simulink model "single_NMM_Adaptive_Controller"  (R2019a)
settings: Solver=ode4  StartTime=0.0  StopTime=10  RelTol=1e-3
PostLoadFcn:
  | ButtonName = questdlg(['Today is ' date newline 'Have a Nice Day' newline...
  |  'The Simulink model was created by Lige on 25-Dec-2019'...
  | newline 'The Author''s Email is lige960103@gmail.com',newline,newline,newline,...
  | 'Would you want the dialog box to be shown when the file is opened again? '], ...
  | 'Open Question', ...
  | 'Yes', 'No', 'Yes');
  | if strcmp(ButtonName,'No')
  | set_param(gcs,'PostLoadFcn','')
  | save_system(gcs)
  | end
  | clear ButtonName
StopFcn:
  | fi=get_param([bdroot '/Show/ref_out'],'Commented');
  | if strcmp(fi,'off')
  | plot(ref_out.Time,ref_out.Data(:,1),ref_out.Time,ref_out.Data(:,2))
  | legend('ref','out')
  | ylabel('y (mV)')
  | xlabel('t')
  | title('Output and Reference')
  | end
  | 
  | fi=get_param([bdroot '/Show/err'],'Commented');
  | if strcmp(fi,'off')
  | figure;
  | plot(err.Time,err.Data)
  | legend('error')
  | ylabel('value (mV)')
  | xlabel('t (s)')
  | title('Tracking Error')
  | end
  | 
  | fi=get_param([bdroot '/Show/Hat_A_and_A'],'Commented');
  | if strcmp(fi,'off')
  | figure;
  | plot(Hat_A_and_A.Time,Hat_A_and_A.Data(:,1),Hat_A_and_A.Time,Hat_A_and_A.Data(:,2))
  | legend('hat A ','A')
  | ylabel('value (mV)')
  | xlabel('t (s)')
  | title('Parameters Estimated')
  | end
  | 
  | fi=get_param([bdroot '/Show/u'],'Commented');
  | if strcmp(fi,'off')
  | figure;
  | plot(u.Time,u.Data)
  | legend('u')
  | ylabel('value (mV)')
  | xlabel('t (s)')
  | title('Control Input')
  | end
undefined symbols (not defined in the file): Single_NMM_Parameters
libraries: simulink x2
settings Model: Creator=Administrator  LastModifiedBy=liuxian
settings DataIOCC: SaveOutput=off  SignalLogging=off  DSMLogging=off  SaveTime=off  ReturnWorkspaceOutputs=off
settings OptimizationCC: DefaultParameterBehavior=Inlined  EnhancedBackFolding=on  PassReuseOutputArgsAs=Individual arguments  OptimizeBlockOrder=speed  DifferentSizesBufferReuse=on  OptimizationCustomize=off
settings DebuggingCC: ParameterTunabilityLossMsg=error
settings SFSimCC: MATLABDynamicMemAlloc=off
settings RTWCC: SystemTargetFile=ert.tlc  TemplateMakefile=ert_default_tmf  GenerateReport=on  IncludeHyperlinkInReport=on  LaunchReport=on  GenerateTraceInfo=on  GenerateTraceReport=on  GenerateTraceReportSl=on  GenerateTraceReportSf=on  GenerateTraceReportEml=on
settings CodeAppCC: ForceParamTrailComments=on  IgnoreCustomStorageClasses=off  OperatorAnnotations=on  SimulinkDataObjDesc=on  SFDataObjDesc=on  InsertBlockDesc=on
settings ERTTargetCC: TargetLangStandard=C99 (ISO)  GenerateSampleERTMain=on  MatFileLogging=on  SupportContinuousTime=on  InlinedParameterPlacement=NonHierarchical  ERTCustomFileTemplate=example_file_process.tlc  ERTFilePackagingFormat=CompactWithDataFile

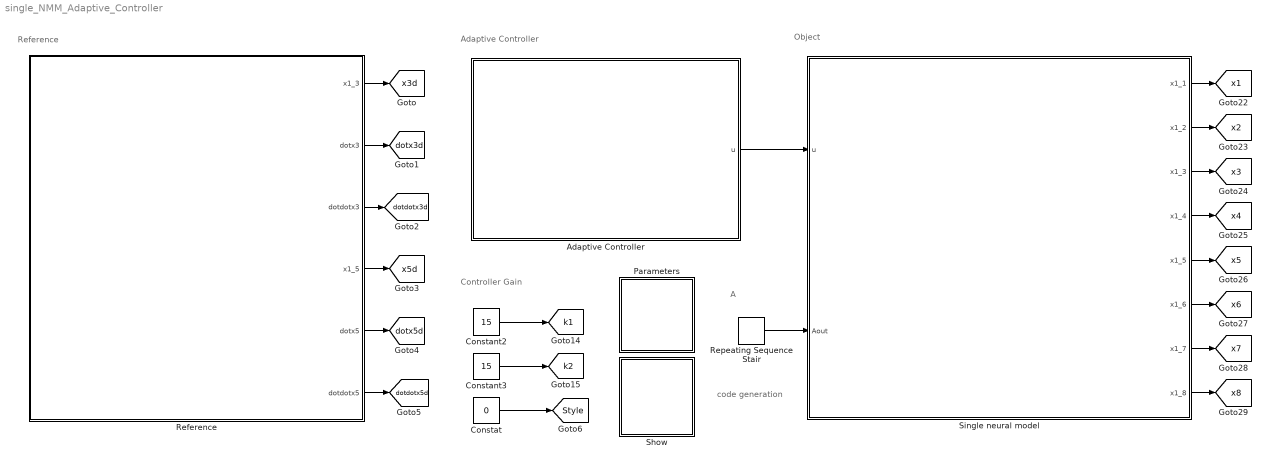
== system single_NMM_Adaptive_Controller ==
  note: code
      | generation
  note: Controller Gain
  note: Adaptive Controller
  note: Reference
  note: Object
  note: A
  Adaptive Controller : Subsystem
      settings: RTWSystemCode=Nonreusable function  RTWFcnNameOpts=Use subsystem name
      mask Display: disp('Adaptive Controller')
  Constant2 : Constant  Value=15
  Constant3 : Constant  Value=15
  Constat : Constant  Value=0  OutDataTypeStr=boolean
  Parameters : Subsystem
      mask Display: disp('Param')
  Reference : Subsystem  mask(Reference  model){AA=Single_NMM_Parameters.Normal_A, B=Single_NMM_Parameters.B, a=Single_NMM_Parameters.a, b1=Single_NMM_Parameters.b, C_1=Single_NMM_Parameters.C1, C_2=Single_NMM_Parameters.C2, C_3=Single_NMM_Parameters.C3, C_4=Single_NMM_Parameters.C4, r=Single_NMM_Parameters.r, e_0=Single_NMM_Parameters.e_0, v_0=Single_NMM_Parameters.v_0, a_d=Single_NMM_Parameters.a_d, SimpleTime=Single_NMM_Parameters.simple_time}
      mask prompts: AA "A"; b1 "b"; C_1 "C1"; C_2 "C2"; C_3 "C3"; C_4 "C4"; e_0 "e0"; v_0 "v0"; a_d "ad"; SimpleTime "Simple Time of P(t)"
      mask help: The block is the mask of the neural mass model (NMM). The parameters(A and B) are average gain, and the parameter A will result in different model output. The parameters (a, a_d and b) is time constant. The parameter (C1-C4) are average number. Three parameters (v_0, e_0 anf r) define a nonlinear function named sigmoid function.
      settings: RTWSystemCode=Nonreusable function  RTWFcnNameOpts=Use subsystem name
      mask Display:
      | port_label('output',1,'x3')
      | port_label('output',2,'dotx3')
      | port_label('output',3,'dotdotx3')
      | port_label('output',4,'x5')
      | port_label('output',5,'dotx5')
      | port_label('output',6,'dotdotx5')
      | disp('Reference Normal Single NMM')
  Repeating Sequence Stair : simulink/Sources/Repeating Sequence Stair  OutValues=[3.25 3.4 3.5 3.6 3.4 ].'  tsamp=2  OutMin=[]  OutMax=[]  OutDataTypeStr=double  OutputDataTypeScalingMode=double  OutDataType=fixdt(0,8)  ConRadixGroup=Best Precision: Vector-wise  OutScaling=2^-12
  Show : Subsystem
      mask Display: disp('Show')
  Single neural model : Subsystem  mask(Mask Single neural model by lige){A_status=off, AA=Single_NMM_Parameters.Abnormal_A, B=Single_NMM_Parameters.B, a=Single_NMM_Parameters.a, b1=Single_NMM_Parameters.b, C_1=Single_NMM_Parameters.C1, C_2=Single_NMM_Parameters.C2, C_3=Single_NMM_Parameters.C3, C_4=Single_NMM_Parameters.C4, r=Single_NMM_Parameters.r, e_0=Single_NMM_Parameters.e_0, v_0=Single_NMM_Parameters.v_0, a_d=Single_NMM_Parameters.a_d, SimpleTime=Single_NMM_Parameters.simple_time}
      mask prompts: A_status "Change A in GUI or input"; AA "A"; b1 "b"; C_1 "C1"; C_2 "C2"; C_3 "C3"; C_4 "C4"; e_0 "e0"; v_0 "v0"; a_d "ad"; SimpleTime "Simple Time of P(t)"
      mask help: The block is the mask of the neural mass model (NMM). The parameters(A and B) are average gain, and the parameter A will result in different model output. The parameters (a, a_d and b) is time constant. The parameter (C1-C4) are average number. Three parameters (v_0, e_0 anf r) define a nonlinear function named sigmoid function.
      settings: RTWSystemCode=Nonreusable function  RTWFcnNameOpts=Use subsystem name
      mask Callback A_status:
      | A_s=get(gcbh,'A_status');
      | block_name=gcb;
      | A_vis=get(gcbh,'MaskVisibilities');
      | str=['port_label(''input'',1,''u'');'...
      | 'port_label(''input'',2,''The port is unvalid'');'...
      | 'port_label(''output'',1,''x_1'');'...
      | 'port_label(''output'',2,''x_2'');'...
      | 'port_label(''output'',3,''x_3'');'...
      | 'port_label(''output'',4,''x_4'');'...
      | 'port_label(''output'',5,''x_5'');'...
      | 'port_label(''output'',6,''x_6'');'...
      | 'port_label(''output'',7,''x_7'');'...
      | 'port_label(''output'',8,''x_8'');disp(''Single NMM'')'];
      | str1=['port_label(''input'',1,''u'');'...
      | 'port_label(''input'',2,''A'');'...
      | 'port_label(''output'',1,''x_1'');'...
      | 'port_label(''output'',2,''x_2'');'...
      | 'port_label(''output'',3,''x_3'');'...
      | 'port_label(''output'',4,''x_4'');'...
      | 'port_label(''output'',5,''x_5'');'...
      | 'port_label(''output'',6,''x_6'');'...
      | 'port_label(''output'',7,''x_7'');'...
      | 'port_label(''output'',8,''x_8'');disp(''Single NMM'')'];
      | if strcmp(A_s,'on')
      |     set(gcbh,'MaskDisplay',str)
      |     A_vis{2}='on';
      |     set_param([block_name '/gain'],'Gain','1');
      |     set_param([block_name '/gaout'],'Gain','0');
      | else
      |     set(gcbh,'MaskDisplay',str1)
      |     A_vis{2}='off';
      |     set_param([block_name '/gain'],'Gain','0');
      |     set_param([block_name '/gaout'],'Gain','1');
      | end
      | set(gcbh,'MaskVisibilities',A_vis)
      mask Display: port_label('input',1,'u');port_label('input',2,'A');port_label('output',1,'x_1');port_label('output',2,'x_2');port_label('output',3,'x_3');port_label('output',4,'x_4');port_label('output',5,'x_5');port_label('output',6,'x_6');port_label('output',7,'x_7');port_label('output',8,'x_8');disp('Single NMM')
  tag scope: Style=global, dotdotx3d=global, dotdotx5d=global, dotx3d=global, dotx5d=global, k1=global, k2=global, x1=global, x2=global, x3=global, x3d=global, x4=global, x5=global, x5d=global, x6=global, x7=global, x8=global
  wires:
  Repeating Sequence Stair/1 -> Single neural model/2(Aout)
  Single neural model/1(x1_1) -> [x1]
  Single neural model/2(x1_2) -> [x2]
  Single neural model/3(x1_3) -> [x3]
  Single neural model/4(x1_4) -> [x4]
  Single neural model/5(x1_5) -> [x5]
  Single neural model/6(x1_6) -> [x6]
  Single neural model/7(x1_7) -> [x7]
  Single neural model/8(x1_8) -> [x8]
  Reference/3(dotdotx3) -> [dotdotx3d]
  Reference/1(x1_3) -> [x3d]
  Reference/2(dotx3) -> [dotx3d]
  Reference/4(x1_5) -> [x5d]
  Reference/5(dotx5) -> [dotx5d]
  Reference/6(dotdotx5) -> [dotdotx5d]
  Constant2/1 -> [k1]
  Constant3/1 -> [k2]
  Adaptive Controller/1(u) -> Single neural model/1(u)
  Constat/1 -> [Style]

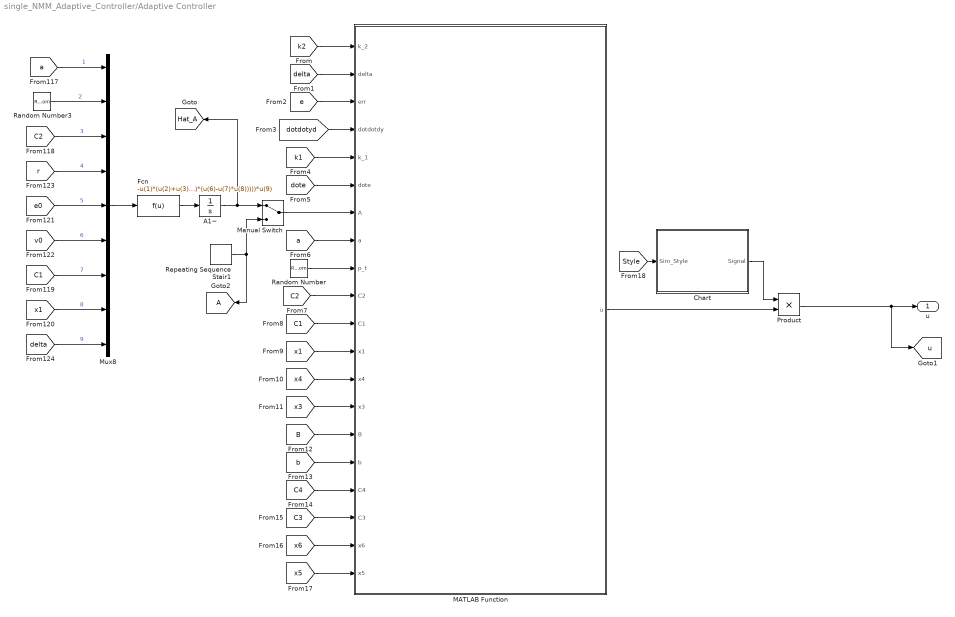
== system single_NMM_Adaptive_Controller/Adaptive Controller ==
  A1~ : Integrator  InitialCondition=3  LimitOutput=on  UpperSaturationLimit=6  LowerSaturationLimit=2
  Chart : Stateflow chart  BlockKeywords=__PRM__SERIALIZED__DATA__:Stateflow Chart,Stateflow Diagram  TreatAsAtomicUnit=on
  Fcn : Fcn  Expr=-u(1)*(u(2)+u(3)*2*u(5)/(1+exp(u(4)*(u(6)-u(7)*u(8)))))*u(9)
  MATLAB Function : MATLAB Function  TreatAsAtomicUnit=on
  Manual Switch : ManualSwitch
  Mux8 : Mux  Inputs=9
  Product : Product
  Random Number : RandomNumber  Mean=90  Variance=30  SampleTime=Single_NMM_Parameters.simple_time
  Random Number3 : RandomNumber  Mean=90  Variance=30  SampleTime=Single_NMM_Parameters.simple_time
  Repeating Sequence Stair1 : simulink/Sources/Repeating Sequence Stair  OutValues=[3.25 3.4 3.5 3.6 3.4 ].'  tsamp=2  OutMin=[]  OutMax=[]  OutDataTypeStr=double  OutputDataTypeScalingMode=double  OutDataType=fixdt(0,8)  ConRadixGroup=Best Precision: Vector-wise  OutScaling=2^-12
  u : Outport
  tag scope: A=global, Hat_A=global, u=global
  wires:
  [x3] -> MATLAB Function/14(x3)
  [C1] -> Mux8/7  "7"
  [v0] -> Mux8/6  "6"
  Repeating Sequence Stair1/1 -> Manual Switch/2, [A]
  Fcn/1 -> A1~/1
  [a] -> MATLAB Function/8(a)
  [k1] -> MATLAB Function/5(k_1)
  [C3] -> MATLAB Function/18(C3)
  A1~/1 -> [Hat_A], Manual Switch/1
  [r] -> Mux8/4  "4"
  [e] -> MATLAB Function/3(err)
  Mux8/1 -> Fcn/1
  [b] -> MATLAB Function/16(b)
  Random Number3/1 -> Mux8/2  "2"
  [x1] -> MATLAB Function/12(x1)
  [k2] -> MATLAB Function/1(k_2)
  [C1] -> MATLAB Function/11(C1)
  [e0] -> Mux8/5  "5"
  [x6] -> MATLAB Function/19(x6)
  [dotdotyd] -> MATLAB Function/4(dotdotdy)
  [delta] -> MATLAB Function/2(delta)
  [a] -> Mux8/1  "1"
  [C2] -> Mux8/3  "3"
  [C2] -> MATLAB Function/10(C2)
  [dote] -> MATLAB Function/6(dote)
  Manual Switch/1 -> MATLAB Function/7(A)
  [C4] -> MATLAB Function/17(C4)
  [x5] -> MATLAB Function/20(x5)
  Product/1 -> [u], u/1
  [x1] -> Mux8/8  "8"
  [delta] -> Mux8/9  "9"
  [B] -> MATLAB Function/15(B)
  Random Number/1 -> MATLAB Function/9(p_t)
  [x4] -> MATLAB Function/13(x4)
  Chart/1(Signal) -> Product/1
  MATLAB Function/1(u) -> Product/2
  [Style] -> Chart/1(Sim_Style)

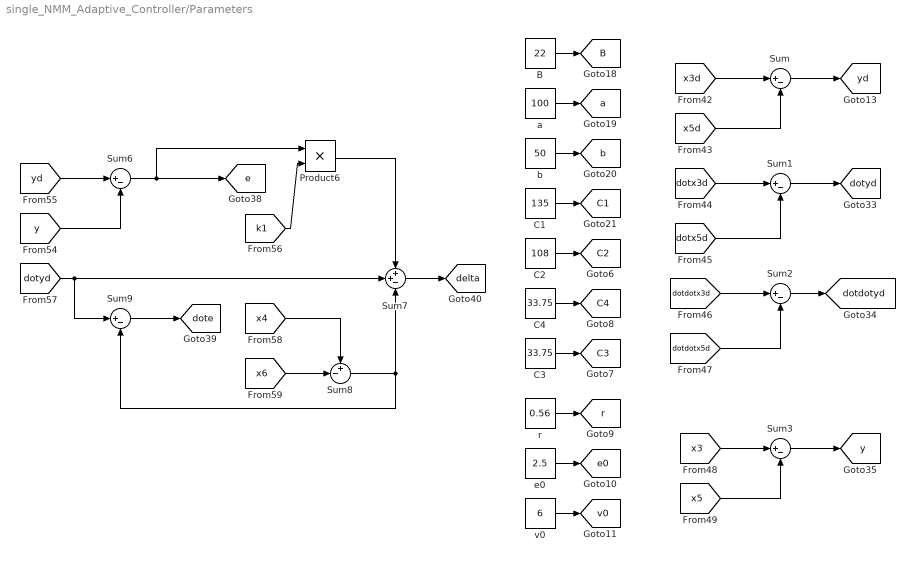
== system single_NMM_Adaptive_Controller/Parameters ==
  B : Constant  Value=22
  C1 : Constant  Value=135
  C2 : Constant  Value=108
  C3 : Constant  Value=33.75
  C4 : Constant  Value=33.75
  Product6 : Product
  Sum{,1..3,6,9} (6 alike) : Sum  Inputs=|+-
  Sum7 : Sum  Inputs=++-
  Sum8 : Sum  Inputs=+-|
  a : Constant  Value=100
  b : Constant  Value=50
  e0 : Constant  Value=2.5
  r : Constant  Value=0.56
  v0 : Constant  Value=6
  tag scope: B=global, C1=global, C2=global, C3=global, C4=global, a=global, b=global, delta=global, dotdotyd=global, dote=global, dotyd=global, e0=global, e=global, r=global, v0=global, y=global, yd=global
  wires:
  [dotx3d] -> Sum1/1
  [dotdotx5d] -> Sum2/2
  Sum9/1 -> [dote]
  [dotx5d] -> Sum1/2
  B/1 -> [B]
  e0/1 -> [e0]
  C2/1 -> [C2]
  [yd] -> Sum6/1
  [dotyd] -> Sum9/1, Sum7/2
  Sum7/1 -> [delta]
  Sum1/1 -> [dotyd]
  a/1 -> [a]
  [dotdotx3d] -> Sum2/1
  Sum/1 -> [yd]
  [k1] -> Product6/2
  Sum6/1 -> Product6/1, [e]
  r/1 -> [r]
  [x5d] -> Sum/2
  Sum8/1 -> Sum7/3, Sum9/2
  C3/1 -> [C3]
  b/1 -> [b]
  [x4] -> Sum8/1
  C4/1 -> [C4]
  [y] -> Sum6/2
  [x3] -> Sum3/1
  Sum2/1 -> [dotdotyd]
  [x6] -> Sum8/2
  Sum3/1 -> [y]
  C1/1 -> [C1]
  v0/1 -> [v0]
  [x5] -> Sum3/2
  Product6/1 -> Sum7/1
  [x3d] -> Sum/1

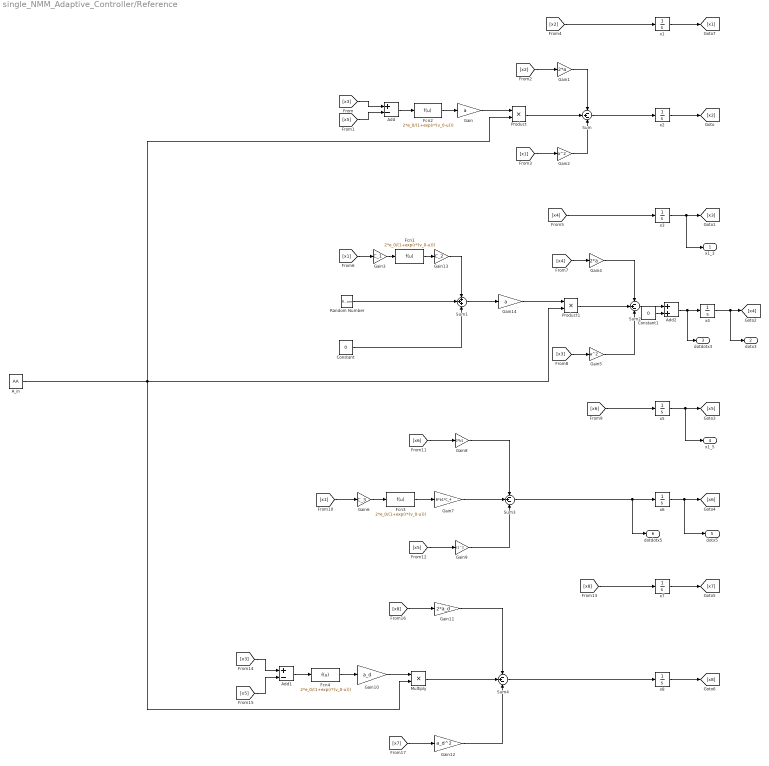
== system single_NMM_Adaptive_Controller/Reference ==
  A_in : Constant  Value=AA
  Add : Sum  Inputs=+-
  Add1 : Sum  Inputs=+-
  Add2 : Sum
  Constant : Constant  Value=0
  Constant1 : Constant  Value=0
  Fcn{1..4} (4 alike) : Fcn  Expr=2*e_0/(1+exp(r*(v_0-u)))
  Gain : Gain  Gain=a
  Gain1 : Gain  Gain=2*a
  Gain10 : Gain  Gain=a_d
  Gain11 : Gain  Gain=2*a_d
  Gain12 : Gain  Gain=a_d^2
  Gain13 : Gain  Gain=C_2
  Gain14 : Gain  Gain=a
  Gain2 : Gain  Gain=a^2
  Gain3 : Gain  Gain=C_1
  Gain4 : Gain  Gain=2*a
  Gain5 : Gain  Gain=a^2
  Gain6 : Gain  Gain=C_3
  Gain7 : Gain  Gain=B*b1*C_4
  Gain8 : Gain  Gain=2*b1
  Gain9 : Gain  Gain=b1^2
  Multiply : Product
  Product : Product
  Product1 : Product
  Random Number : RandomNumber  Mean=90  Variance=30  SampleTime=SimpleTime
  Sum{,2..4} (4 alike) : Sum  Inputs=-+-
  Sum1 : Sum  Inputs=3
  x{1..8} (8 alike) : Integrator
  x1_3 : Outport
  dotx3 : Outport  Port=2
  dotdotx3 : Outport  Port=3
  x1_5 : Outport  Port=4
  dotx5 : Outport  Port=5
  dotdotx5 : Outport  Port=6
  wires:
  Gain/1 -> Product/1
  Gain12/1 -> Sum4/3
  Gain2/1 -> Sum/3
  Random Number/1 -> Sum1/2
  Gain11/1 -> Sum4/1
  [x5] -> Add1/2
  [x1] -> Gain6/1
  Gain13/1 -> Sum1/1
  [x6] -> Gain8/1
  [x6] -> x5/1
  [x3] -> Gain5/1
  Sum/1 -> x2/1
  [x1] -> Gain2/1
  [x4] -> Gain4/1
  Sum2/1 -> Add2/1
  Fcn3/1 -> Gain7/1
  [x8] -> x7/1
  A_in/1 -> Product/2, Multiply/2, Product1/2
  [x2] -> Gain1/1
  Multiply/1 -> Sum4/2
  Gain8/1 -> Sum3/1
  [x2] -> x1/1
  Product1/1 -> Sum2/2
  Gain14/1 -> Product1/1
  Gain6/1 -> Fcn3/1
  Product/1 -> Sum/2
  Add/1 -> Fcn2/1
  Gain9/1 -> Sum3/3
  x5/1 -> [x5], x1_5/1
  [x4] -> x3/1
  x3/1 -> [x3], x1_3/1
  [x3] -> Add/1
  [x8] -> Gain11/1
  Fcn1/1 -> Gain13/1
  [x5] -> Add/2
  Gain5/1 -> Sum2/3
  [x3] -> Add1/1
  Gain7/1 -> Sum3/2
  Add1/1 -> Fcn4/1
  [x5] -> Gain9/1
  [x7] -> Gain12/1
  Sum3/1 -> dotdotx5/1, x6/1
  x1/1 -> [x1]
  x6/1 -> [x6], dotx5/1
  Gain1/1 -> Sum/1
  [x1] -> Gain3/1
  Gain4/1 -> Sum2/1
  x2/1 -> [x2]
  Fcn2/1 -> Gain/1
  Add2/1 -> dotdotx3/1, x4/1
  x4/1 -> [x4], dotx3/1
  x8/1 -> [x8]
  x7/1 -> [x7]
  Gain10/1 -> Multiply/1
  Gain3/1 -> Fcn1/1
  Sum1/1 -> Gain14/1
  Sum4/1 -> x8/1
  Constant1/1 -> Add2/2
  Constant/1 -> Sum1/3
  Fcn4/1 -> Gain10/1

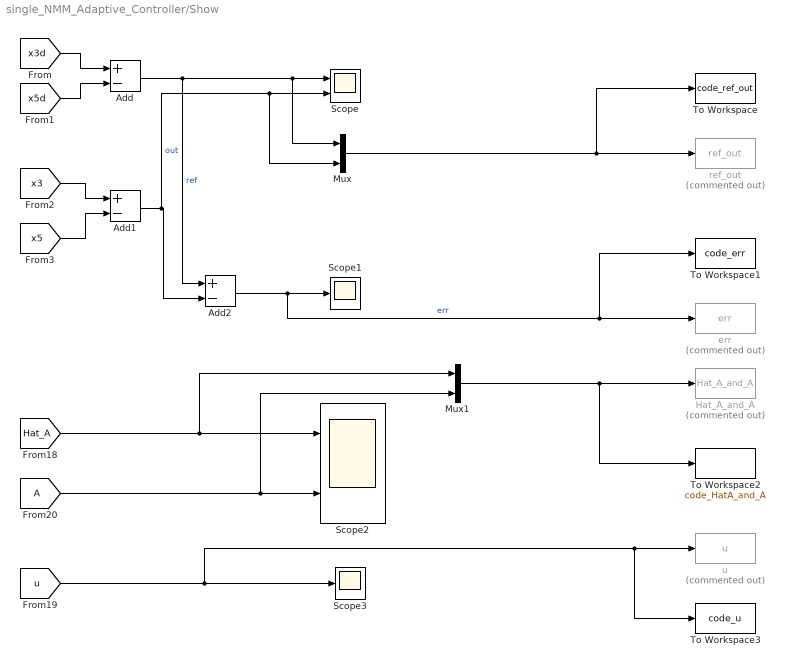
== system single_NMM_Adaptive_Controller/Show ==
  Add : Sum  Inputs=+-
  Add1 : Sum  Inputs=+-
  Add2 : Sum  Inputs=+-
  Hat_A_and_A : ToWorkspace  Commented=on  VariableName=Hat_A_and_A  SaveFormat=Timeseries  SampleTime=-1
  Mux : Mux  Inputs=2
  Mux1 : Mux  Inputs=2
  Scope : Scope  NumInputPorts=2
  Scope1 : Scope
  Scope2 : Scope  NumInputPorts=2
  Scope3 : Scope
  To Workspace : ToWorkspace  VariableName=code_ref_out  SaveFormat=Structure With Time  SampleTime=-1
  To Workspace1 : ToWorkspace  VariableName=code_err  SaveFormat=Structure With Time  SampleTime=-1
  To Workspace2 : ToWorkspace  VariableName=code_HatA_and_A  SaveFormat=Structure With Time  SampleTime=-1
  To Workspace3 : ToWorkspace  VariableName=code_u  SaveFormat=Structure With Time  SampleTime=-1
  err : ToWorkspace  Commented=on  VariableName=err  SaveFormat=Timeseries  SampleTime=-1
  ref_out : ToWorkspace  Commented=on  VariableName=ref_out  SaveFormat=Timeseries  SampleTime=-1
  u : ToWorkspace  Commented=on  VariableName=u  SaveFormat=Timeseries  SampleTime=-1
  wires:
  [x3d] -> Add/1
  [x5d] -> Add/2
  [x3] -> Add1/1
  [x5] -> Add1/2
  Add1/1 -> Mux/2, Scope/2, Add2/2  "out"
  Add/1 -> Add2/1, Mux/1, Scope/1  "ref"
  Add2/1 -> err/1, To Workspace1/1, Scope1/1  "err"
  [Hat_A] -> Mux1/1, Scope2/1
  [A] -> Mux1/2, Scope2/2
  Mux1/1 -> Hat_A_and_A/1, To Workspace2/1
  Mux/1 -> To Workspace/1, ref_out/1
  [u] -> To Workspace3/1, u/1, Scope3/1

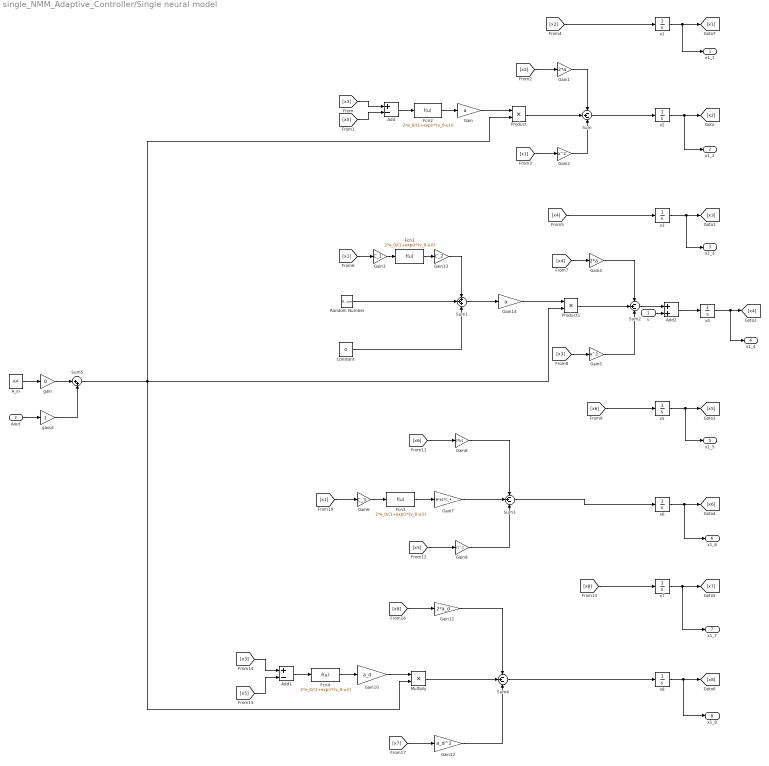
== system single_NMM_Adaptive_Controller/Single neural model ==
  u : Inport
  Aout : Inport  Port=2
  A_in : Constant  Value=AA
  Add : Sum  Inputs=+-
  Add1 : Sum  Inputs=+-
  Add2 : Sum
  Constant : Constant  Value=0
  Fcn{1..4} (4 alike) : Fcn  Expr=2*e_0/(1+exp(r*(v_0-u)))
  Gain : Gain  Gain=a
  Gain1 : Gain  Gain=2*a
  Gain10 : Gain  Gain=a_d
  Gain11 : Gain  Gain=2*a_d
  Gain12 : Gain  Gain=a_d^2
  Gain13 : Gain  Gain=C_2
  Gain14 : Gain  Gain=a
  Gain2 : Gain  Gain=a^2
  Gain3 : Gain  Gain=C_1
  Gain4 : Gain  Gain=2*a
  Gain5 : Gain  Gain=a^2
  Gain6 : Gain  Gain=C_3
  Gain7 : Gain  Gain=B*b1*C_4
  Gain8 : Gain  Gain=2*b1
  Gain9 : Gain  Gain=b1^2
  Multiply : Product
  Product : Product
  Product1 : Product
  Random Number : RandomNumber  Mean=90  Variance=30  SampleTime=SimpleTime
  Sum{,2..4} (4 alike) : Sum  Inputs=-+-
  Sum1 : Sum  Inputs=3
  Sum5 : Sum  Inputs=|++
  gain : Gain  Gain=0
  gaout : Gain
  x{1..8} (8 alike) : Integrator
  x1_1 : Outport
  x1_2 : Outport  Port=2
  x1_3 : Outport  Port=3
  x1_4 : Outport  Port=4
  x1_5 : Outport  Port=5
  x1_6 : Outport  Port=6
  x1_7 : Outport  Port=7
  x1_8 : Outport  Port=8
  wires:
  gaout/1 -> Sum5/2
  gain/1 -> Sum5/1
  A_in/1 -> gain/1
  Aout/1 -> gaout/1
  Sum5/1 -> Product1/2, Multiply/2, Product/2
  Gain10/1 -> Multiply/1
  Multiply/1 -> Sum4/2
  Gain14/1 -> Product1/1
  Product1/1 -> Sum2/2
  Product/1 -> Sum/2
  Gain/1 -> Product/1
  Sum4/1 -> x8/1
  x7/1 -> x1_7/1, [x7]
  [x1] -> Gain6/1
  Gain9/1 -> Sum3/3
  Gain11/1 -> Sum4/1
  Gain13/1 -> Sum1/1
  [x6] -> x5/1
  [x6] -> Gain8/1
  Add/1 -> Fcn2/1
  [x3] -> Gain5/1
  x8/1 -> x1_8/1, [x8]
  Sum/1 -> x2/1
  x4/1 -> x1_4/1, [x4]
  Gain3/1 -> Fcn1/1
  Sum1/1 -> Gain14/1
  Gain5/1 -> Sum2/3
  [x2] -> x1/1
  x5/1 -> x1_5/1, [x5]
  [x5] -> Add/2
  Gain12/1 -> Sum4/3
  x2/1 -> x1_2/1, [x2]
  [x8] -> Gain11/1
  Fcn1/1 -> Gain13/1
  [x3] -> Add/1
  [x8] -> x7/1
  [x1] -> Gain3/1
  Gain4/1 -> Sum2/1
  [x7] -> Gain12/1
  [x4] -> Gain4/1
  Gain2/1 -> Sum/3
  [x2] -> Gain1/1
  x3/1 -> x1_3/1, [x3]
  [x5] -> Gain9/1
  Random Number/1 -> Sum1/2
  x6/1 -> x1_6/1, [x6]
  Gain1/1 -> Sum/1
  Gain7/1 -> Sum3/2
  x1/1 -> x1_1/1, [x1]
  Fcn3/1 -> Gain7/1
  [x4] -> x3/1
  [x1] -> Gain2/1
  Fcn2/1 -> Gain/1
  Gain8/1 -> Sum3/1
  Gain6/1 -> Fcn3/1
  [x5] -> Add1/2
  Constant/1 -> Sum1/3
  [x3] -> Add1/1
  Add2/1 -> x4/1
  Sum2/1 -> Add2/1
  u/1 -> Add2/2
  Sum3/1 -> x6/1
  Add1/1 -> Fcn4/1
  Fcn4/1 -> Gain10/1

== matlab function single_NMM_Adaptive_Controller/Adaptive Controller/MATLAB Function ==
  data: k_2 input; u output; delta input; err input; dotdotdy input; k_1 input; dote input; A input; a input; p_t input; C2 input; C1 input; x1 input; x4 input; x3 input; B input; b input; C4 input; C3 input; x6 input; x5 input
function u = adptive_controller(k_2,delta,err,dotdotdy,k_1,dote,A,a,p_t,C2,C1,x1,x4,x3,B,b,C4,C3,x6,x5)
%codergen
u=k_2*delta+err+dotdotdy+k_1*dote-A*a*(p_t+C2*2*2.5/(1+exp(0.56*(6-C1*x1))))...
    +2*a*x4+a^2*x3+B*b*C4*2*2.5/(1+exp(0.56*(6-C3*x1)))-2*b*x6-b^2*x5;

== stateflow chart single_NMM_Adaptive_Controller/Adaptive Controller/Chart ==
  state All
    en:
    Signal = true;
  state Uncontroll
    en:
    Signal=false;
  state Controll
    en:
    Signal = true;
  state Uncontroll1
    en:
    Signal=false;
  state Controll1
    en:
    Signal = true;
  state Uncontroll2
    en:
    Signal=false;
  state Controll4
    en:
    Signal = true;
  state Uncontroll4
    en:
    Signal=false;
  state Controll3
    en:
    Signal = true;
  state Uncontroll3
    en:
    Signal=false;
  state Controll2
    en:
    Signal = true;
  (default) -> Uncontroll [order 1] : [Sim_Style == 0]
  (default) -> All [order 2]
  Uncontroll1 -> Controll1 : after(0.815,sec)
  Uncontroll -> Controll : after(1.1,sec)
  Controll -> Uncontroll1 : after(0.9,sec)
  Controll1 -> Uncontroll2 : after(1.185,sec)
  Uncontroll2 -> Controll2 : after(0.831,sec)
  Uncontroll4 -> Controll4 : after(1.031,sec)
  Controll2 -> Uncontroll3 : after(1.169,sec)
  Controll3 -> Uncontroll4 : after(1.05,sec)
  Uncontroll3 -> Controll3 : after(.95,sec)
  data: Sim_Style input boolean; Signal output boolean
